simulink model "L400_airframe"  (R2024b)
settings: Solver=FixedStepAuto  StartTime=0  StopTime=10  FixedStep=5/1000  RelTol=1e-3
values from neighbouring files (symbols this model uses):
  db =     [L400_airframe_data.mat]
undefined symbols (not defined in the file or in its folder): lambda
libraries: aerolibconvert2 x16, simulink x6, matrix_library x4, aerolibactuator x2, shared6dof x1, aerolibtransform2 x1
(part 1 of 4)
settings Model: DataDictionary=nextpilot_datadict.sldd  PauseTimes=10  Creator=zhanfuyu  LastModifiedBy=CETCA
settings OptimizationCC: BlockReduction=off  OptimizeBlockIOStorage=off  BufferReuse=off  ReuseModelBlockBuffer=off
settings DebuggingCC: AlgebraicLoopMsg=none
settings RTWCC: GPUComputeCapability=3.5

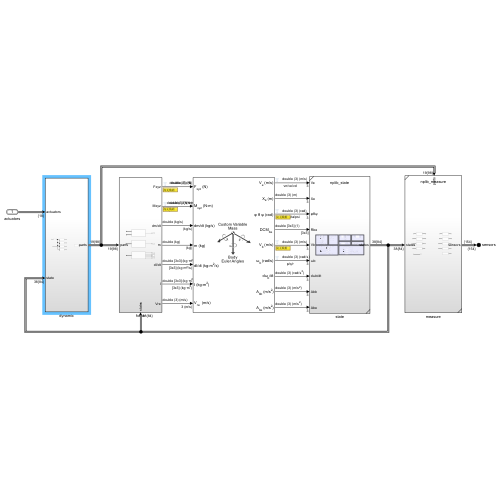
[thumbnail: Simulink's stored preview of the top-level diagram]
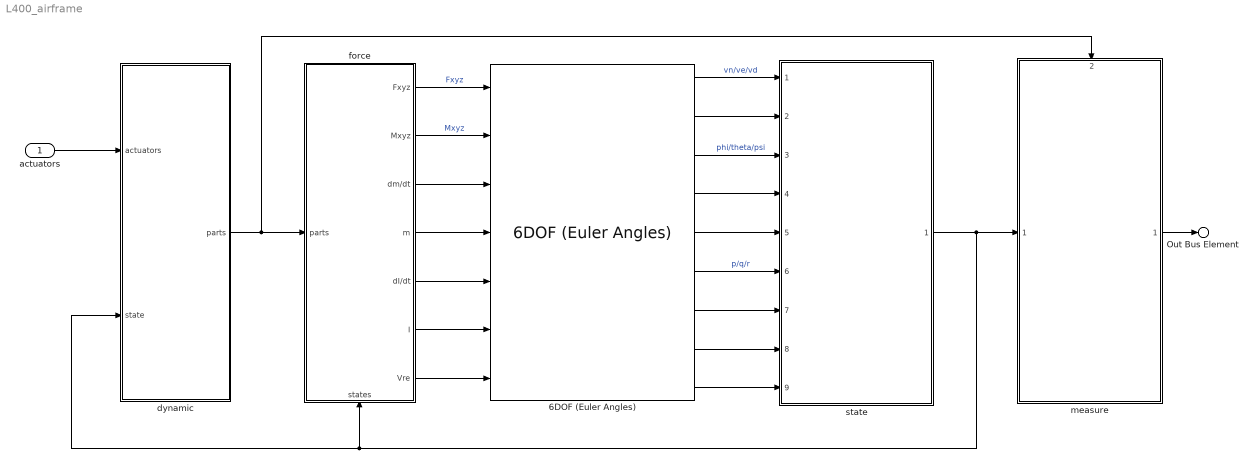
== system L400_airframe ==
  actuators : Inport  OutDataTypeStr=Bus: actuator_outputs_s
  6DOF (Euler Angles) : shared6dof/6DOF (Euler Angles)  units=Metric (MKS)  mtype=Custom Variable  rep=Euler Angles  xme_0=[0 0 0]  Vm_0=INIT_U_V_W  eul_0=INIT_PHI_THETA_PSI  pm_0=INIT_P_Q_R  mass_0=db.mass.empty_weight  mass_e=0.5  mass_f=2.0  inertia=db.mass.empty_inertia  inertia_e=eye(3)  inertia_f=2*eye(3)  k_quat=1.0  vre_flag=on  abi_flag=on  aMode=0  xme_statename=''  Vm_statename=''  eul_statename=''  quat_statename=''  pm_statename=''  mass_statename=''
  dynamic : Subsystem
  force : Subsystem
      settings: PortSchema="{\"entries\":[{\"content\":{\"sides\":[{\"content\":{\"connectorIds\":[\"In1\"]},\"type\":\"ConnectorPlacement.EquallySpacedRectSide\",\"uuid\":\"0db1562e-dce2-4925-bed5-09f9d5b35c44\"},{\"content\":{\"connectorIds\":[\"Out1\",\"Out2\",\"Out3\",\"Out4\",\"Out5\",\"Out6\",\"Out7\"],\"side\":\"RIGHT\"},\"type\":\"ConnectorPlacement.EquallySpacedRectSide\",\"uuid\":\"7a0bc065-1050-4432-a746-8dc7f5e520af\"},{\"content\":{\"side\":\"TOP\"},\"type\":\"ConnectorPlacement.EquallySpacedRectSide\",\"uuid\":\"d0d45c02-cab6-4ab9-ab13-36238f6ff9ea\"},{\"content\":{\"connectorIds\":[\"In2\"],\"side\":\"BOTTOM\"},\"type\":\"ConnectorPlacement.EquallySpacedRectSide\",\"uuid\":\"de54a8ab-f9a4-4296-8b1a-e4e0d752d409\"}]},\"type\":\"ConnectorPlacement.EquallySpacedConnector\",\"uuid\":\"66df0e54-381c-4367-9374-a8940782ebe2\"}],\"packageUris\":[\"http://schema.mathworks.com/mf0/Connector/R2020b\"],\"version\":\"1.0\"}"
  measure : Subsystem  ReferencedSubsystem=nplib_measure
      settings: PortSchema="{\"entries\":[{\"content\":{\"sides\":[{\"content\":{\"connectorIds\":[\"In1\"]},\"type\":\"ConnectorPlacement.EquallySpacedRectSide\",\"uuid\":\"2aab4ced-4e9b-468f-a65b-188f78e0a938\"},{\"content\":{\"connectorIds\":[\"Out1\"],\"side\":\"RIGHT\"},\"type\":\"ConnectorPlacement.EquallySpacedRectSide\",\"uuid\":\"584354fc-f574-4b95-9f8d-a092ecf8eb84\"},{\"content\":{\"connectorIds\":[\"In2\"],\"side\":\"TOP\"},\"type\":\"ConnectorPlacement.EquallySpacedRectSide\",\"uuid\":\"a8f99752-a379-47dc-8675-e6d7e7135bd2\"}]},\"type\":\"ConnectorPlacement.EquallySpacedConnector\",\"uuid\":\"3b032698-2e8e-44bf-976a-546e344c3b42\"}],\"packageUris\":[\"http://schema.mathworks.com/mf0/Connector/R2020b\"],\"version\":\"1.0\"}"
  state : Subsystem  ReferencedSubsystem=nplib_state
  Out Bus Element : Outport  PortName=sensors
  wires:
  state/1 -> dynamic/2(state), force/2(states), measure/1
  measure/1 -> Out Bus Element/1
  actuators/1 -> dynamic/1(actuators)
  6DOF (Euler Angles)/1 -> state/1  "vn/ve/vd"
  6DOF (Euler Angles)/2 -> state/2
  6DOF (Euler Angles)/3 -> state/3  "phi/theta/psi"
  6DOF (Euler Angles)/4 -> state/4
  6DOF (Euler Angles)/5 -> state/5
  6DOF (Euler Angles)/6 -> state/6  "p/q/r"
  6DOF (Euler Angles)/7 -> state/7
  6DOF (Euler Angles)/8 -> state/8
  dynamic/1(parts) -> measure/2, force/1(parts)
  force/4(m) -> 6DOF (Euler Angles)/4
  force/6(I) -> 6DOF (Euler Angles)/6
  force/3(dm/dt) -> 6DOF (Euler Angles)/3
  force/5(dI/dt) -> 6DOF (Euler Angles)/5
  force/7(Vre) -> 6DOF (Euler Angles)/7
  6DOF (Euler Angles)/9 -> state/9
  force/1(Fxyz) -> 6DOF (Euler Angles)/1  "Fxyz"
  force/2(Mxyz) -> 6DOF (Euler Angles)/2  "Mxyz"

== system L400_airframe/dynamic ==
  Bus Element In1 : Inport  PortName=actuators
  Bus Element In : Inport  Port=2  PortName=state
  " propulsion" : Subsystem
  Subsystem : Subsystem
  aerodynamic : Subsystem
  battery : Subsystem
  landgear : Subsystem  Variant=on  VariantControlMode=label  LabelModeActiveChoice=Simple
  payload : Subsystem
  Bus Element Out : Outport  PortName=parts  Element=aerody
  Bus Element Out1 : Outport  PortName=parts  Element=engine
  Bus Element Out2 : Outport  PortName=parts  Element=landgear
  Bus Element Out3 : Outport  PortName=parts  Element=payload
  Bus Element Out4 : Outport  PortName=parts  Element=battery
  wires:
  Bus Element In1/1 -> Subsystem/1(actuators)
  Subsystem/1(command) -> landgear/1(cmd), payload/1(cmd), " propulsion"/1(cmd), aerodynamic/1(cmd)
  aerodynamic/1(aerody) -> Bus Element Out/1
  " propulsion"/1(engine) -> Bus Element Out1/1
  landgear/1(landgear) -> Bus Element Out2/1
  payload/1(payload) -> Bus Element Out3/1
  battery/1(battery) -> Bus Element Out4/1
  Bus Element In/1 -> landgear/2(state), payload/2(state), aerodynamic/2(state), " propulsion"/2(state)

== system L400_airframe/force ==
  BusElementIn : Inport  PortName=parts
  BusElementIn1 : Inport  PortName=parts
  BusElementIn2 : Inport  PortName=parts
  BusElementIn3 : Inport  Port=2  PortName=states
  Force : Subsystem
  Mass : Subsystem
  Moment : Subsystem
  Fxyz : Outport
  Mxyz : Outport  Port=2
  dm/dt : Outport  Port=3
  m : Outport  Port=4
  dI/dt : Outport  Port=5
  I : Outport  Port=6
  Vre : Outport  Port=7
  wires:
  Force/1(Fxyz) -> Fxyz/1
  BusElementIn/1 -> Force/1(parts)
  BusElementIn1/1 -> Moment/1(parts)
  BusElementIn2/1 -> Mass/1(parts)
  Mass/1(dM/dt) -> dm/dt/1
  Mass/2(M) -> m/1
  Mass/3(dI/dt) -> dI/dt/1
  Mass/4(I) -> I/1
  Mass/5(Vre) -> Vre/1
  Moment/1(Mxyz) -> Mxyz/1
  BusElementIn3/1 -> Force/2(state)

== system L400_airframe/dynamic/ propulsion ==
  Bus Element In : Inport  PortName=cmd  Element=DTLO
  Bus Element In2 : Inport  PortName=cmd  Element=DTLI
  Bus Element In3 : Inport  PortName=cmd  Element=DTRI
  Bus Element In4 : Inport  PortName=cmd  Element=DTRO
  BusElementIn : Inport  Port=2  PortName=state  Element=environ.atmosphere.rho
  BusElementIn1 : Inport  Port=2  PortName=state  Element=aircraft.airdata.vax_vay_vaz
  BusElementIn2 : Inport  Port=2  PortName=state  Element=aircraft.airdata.qbar
  Constant1 : Constant  Value=db.motor.setup_position
  Constant2 : Constant  Value=db.motor.setup_angle
  Constant3 : Constant  Value=db.motor.rotation
  Data Type Conversion : DataTypeConversion  SaturateOnIntegerOverflow=off  RndMeth=Floor
  Dot Product : DotProduct  OutDataTypeStr=Inherit: Inherit via internal rule
  For Each Subsystem : Subsystem  TreatAsAtomicUnit=on
  Gain2 : Gain  Gain=db.aerody.Sref
  Linear Second-Order Actuator : aerolibactuator/Linear Second-Order Actuator  Commented=through  wn_fin=1  z_fin=0.3  fin_act_0=0  fin_act_vel=0
  Mux : Mux
  Product : Product  Inputs=*/
  Signal Specification : SignalSpecification  Unit=m
  Sqrt : Sqrt
  Sum3 : Sum  Inputs=1  CollapseMode=Specified dimension  CollapseDim=2
  Transpose3 : Math  Operator=transpose
  Bus Element Out2 : Outport  PortName=engine  Element=state.rpm
  Bus Element Out3 : Outport  PortName=engine  Element=state.power
  Bus Element Out : Outport  PortName=engine  Element=Fxyz
  Bus Element Out1 : Outport  PortName=engine  Element=Mxyz
  Bus Element Out4 : Outport  PortName=engine  Element=Pxyz
  tag scope: TC=global
  wires:
  Bus Element In3/1 -> Mux/3
  Bus Element In2/1 -> Mux/2
  Bus Element In4/1 -> Mux/4
  Bus Element In/1 -> Mux/1
  Mux/1 -> Data Type Conversion/1
  Constant3/1 -> For Each Subsystem/3(rotation)
  For Each Subsystem/1(thrust) -> Sum3/1, Bus Element Out/1
  For Each Subsystem/2(moment) -> Bus Element Out1/1
  For Each Subsystem/3(power) -> Bus Element Out3/1
  Linear Second-Order Actuator/1 -> For Each Subsystem/1(rpm), Bus Element Out2/1  "rpm"
  Constant1/1 -> Transpose3/1
  BusElementIn/1 -> For Each Subsystem/5(rho)
  BusElementIn1/1 -> For Each Subsystem/4(Va)
  Transpose3/1 -> Signal Specification/1
  Constant2/1 -> For Each Subsystem/2(angle)
  Sum3/1 -> Dot Product/2, Dot Product/1
  Dot Product/1 -> Sqrt/1
  Sqrt/1 -> Product/1
  Product/1 -> [TC]
  BusElementIn2/1 -> Gain2/1
  Gain2/1 -> Product/2
  Data Type Conversion/1 -> Linear Second-Order Actuator/1
  Signal Specification/1 -> Bus Element Out4/1

== system L400_airframe/dynamic/Subsystem ==
  Bus Element In1 : Inport  PortName=actuators  Element=output
  Constant : Constant  Value=false
  Data Type Conversion : DataTypeConversion  SaturateOnIntegerOverflow=off  RndMeth=Floor
  Data Type Conversion1 : DataTypeConversion  SaturateOnIntegerOverflow=off  RndMeth=Floor
  Demux : Demux  Outputs=16
  Bus Element Out1 : Outport  PortName=command  Element=DTLO
  Bus Element Out2 : Outport  PortName=command  Element=DTLI
  Bus Element Out3 : Outport  PortName=command  Element=DTRI
  Bus Element Out4 : Outport  PortName=command  Element=DTRO
  Bus Element Out5 : Outport  PortName=command  Element=DFLO
  Bus Element Out6 : Outport  PortName=command  Element=DFLI
  Bus Element Out7 : Outport  PortName=command  Element=DFRI
  Bus Element Out8 : Outport  PortName=command  Element=DFRO
  Bus Element Out9 : Outport  PortName=command  Element=DAL
  Bus Element Out10 : Outport  PortName=command  Element=DAR
  Bus Element Out11 : Outport  PortName=command  Element=DEL
  Bus Element Out12 : Outport  PortName=command  Element=DEM
  Bus Element Out13 : Outport  PortName=command  Element=DER
  Bus Element Out14 : Outport  PortName=command  Element=DRuder
  Bus Element Out15 : Outport  PortName=command  Element=DBrake
  Bus Element Out16 : Outport  PortName=command  Element=DWheel
  Bus Element Out17 : Outport  PortName=command  Element=Dpayload
  wires:
  Bus Element In1/1 -> Demux/1
  Demux/1 -> Bus Element Out1/1
  Demux/2 -> Bus Element Out2/1
  Demux/3 -> Bus Element Out3/1
  Demux/4 -> Bus Element Out4/1
  Demux/5 -> Bus Element Out5/1
  Demux/6 -> Bus Element Out6/1
  Demux/7 -> Bus Element Out7/1
  Demux/8 -> Bus Element Out8/1
  Demux/9 -> Bus Element Out9/1
  Demux/10 -> Bus Element Out10/1
  Demux/11 -> Bus Element Out11/1
  Demux/12 -> Bus Element Out12/1
  Demux/13 -> Bus Element Out13/1
  Demux/14 -> Bus Element Out14/1
  Demux/15 -> Data Type Conversion1/1
  Demux/16 -> Data Type Conversion/1
  Constant/1 -> Bus Element Out17/1
  Data Type Conversion/1 -> Bus Element Out16/1
  Data Type Conversion1/1 -> Bus Element Out15/1

== system L400_airframe/dynamic/aerodynamic ==
  BusElementIn4 : Inport  PortName=cmd
  Bus Element In1 : Inport  Port=2  PortName=state
  actuator : Subsystem
  aerodynamics : Subsystem
  Bus Element Out1 : Outport  PortName=aerody
  wires:
  BusElementIn4/1 -> actuator/1(command)
  Bus Element In1/1 -> aerodynamics/2(state)
  actuator/1(surface) -> aerodynamics/1(surface)
  aerodynamics/1(aerody) -> Bus Element Out1/1

== system L400_airframe/dynamic/battery ==
  note: 50A放电曲线
  note: 电机的功耗
  Constant : Constant  Value=db.battery.capacity
  Constant1 : Constant  Value=db.battery.other_power
  Constant2 : Constant  Value=0
  Gain : Gain  Gain=1/3600/1000
  Integrator : Integrator
  Polynomial : Polyval  Coefs=db.battery.discharge_curve
  Product : Product  Inputs=/*
  Saturation : Saturate  UpperLimit=db.battery.max_discharge  LowerLimit=0
  Sum : Sum  Inputs=|+-
  Sum1 : Sum  Inputs=|++
  Bus Element Out : Outport  PortName=battery  Element=voltage
  Bus Element Out1 : Outport  PortName=battery  Element=soc
  wires:
  Constant/1 -> Product/1, Sum/1
  Integrator/1 -> Gain/1
  Sum/1 -> Polynomial/1, Product/2
  Product/1 -> Bus Element Out1/1
  Polynomial/1 -> Bus Element Out/1
  Gain/1 -> Saturation/1
  Saturation/1 -> Sum/2
  Constant1/1 -> Sum1/1
  Constant2/1 -> Sum1/2
  Sum1/1 -> Integrator/1

== system L400_airframe/dynamic/landgear ==
  note: 1) Add Subsystem or Model blocks as valid variant choices.
      | 2) You cannot connect blocks at this level. At simulation, connectivity is automatically
      | determined, based on the active variant and port name matching.
  cmd : Inport
  state : Inport  Port=2
  Complete : Subsystem  VariantControl=Complete
  Hold : Subsystem  VariantControl=Hold
  Simple : Subsystem  VariantControl=Simple
  landgear : Outport

== system L400_airframe/dynamic/payload ==
  BusElementIn2 : Inport  PortName=cmd  Element=Dpayload
  BusElementIn : Inport  Port=2  PortName=state  Element=aircraft.attitude.phi_theta_psi
  Angle Conversion : aerolibconvert2/Angle Conversion  IU=rad  OU=deg
  Constant : Constant  Value=db.payload.init_mass
  Constant2 : Constant  Commented=on  Value=db.mass.ref_cog
  Constant3 : Constant  Commented=on  Value=[0 0 0]
  Constant4 : Constant  Value=db.payload.spray_speed
  Constant7 : Constant  Value=0
  Integrator : Integrator  LimitOutput=on  UpperSaturationLimit=db.payload.init_mass  LowerSaturationLimit=0
  Selector : Selector  InputPortWidth=3  IndexOptions=Index vector (dialog)  Indices=2  OutputSizes=1
  Subsystem : Subsystem
  Sum : Sum  Inputs=|+-
  Switch : Switch  Criteria=u2 > Threshold  SaturateOnIntegerOverflow=off  InputSameDT=off
  Bus Element Out : Outport  PortName=payload  Element=Fxyz
  Bus Element Out1 : Outport  PortName=payload  Element=Mxyz
  Bus Element Out2 : Outport  PortName=payload  Element=mass
  Bus Element Out3 : Outport  PortName=payload  Element=inertia
  Bus Element Out4 : Outport  PortName=payload  Element=cog
  Bus Element Out5 : Outport  PortName=payload  Element=Pxyz
  wires:
  Constant2/1 -> Bus Element Out5/1
  Constant3/1 -> Bus Element Out/1, Bus Element Out1/1
  Constant/1 -> Sum/1
  Sum/1 -> Bus Element Out2/1, Subsystem/1(mass)
  BusElementIn/1 -> Selector/1
  Selector/1 -> Angle Conversion/1
  BusElementIn2/1 -> Switch/2
  Constant4/1 -> Switch/1
  Switch/1 -> Integrator/1
  Constant7/1 -> Switch/3
  Integrator/1 -> Sum/2
  Subsystem/2(inertia) -> Bus Element Out3/1
  Angle Conversion/1 -> Subsystem/2(theta)
  Subsystem/1(cog) -> Bus Element Out4/1

== system L400_airframe/force/Force ==
  BusElementIn1 : Inport  PortName=parts  Element=aerody.Fxyz
  BusElementIn2 : Inport  PortName=parts  Element=engine.Fxyz
  BusElementIn3 : Inport  PortName=parts  Element=landgear.Fxyz
  BusElementIn4 : Inport  Port=2  PortName=state  Element=environ.gravity.gx_gy_gz
  Product : Product
  Reshape : Reshape
  Reshape1 : Reshape
  Sum : Sum  Inputs=4
  Sum1 : Sum  Inputs=1  CollapseMode=Specified dimension  CollapseDim=2
  Sum2 : Sum  Inputs=+-|
  Sum3 : Sum  Inputs=1  CollapseMode=Specified dimension  CollapseDim=2
  Fxyz : Outport
  tag scope: Fxyz_no_ground=global
  wires:
  BusElementIn2/1 -> Sum3/1
  BusElementIn1/1 -> Sum/2
  Sum/1 -> Sum2/1, Fxyz/1
  [mass] -> Product/1
  Sum3/1 -> Reshape/1
  Reshape/1 -> Sum/3
  BusElementIn3/1 -> Sum1/1
  BusElementIn4/1 -> Product/2
  Sum1/1 -> Reshape1/1
  Reshape1/1 -> Sum/4, Sum2/2
  Product/1 -> Sum/1
  Sum2/1 -> [Fxyz_no_ground]

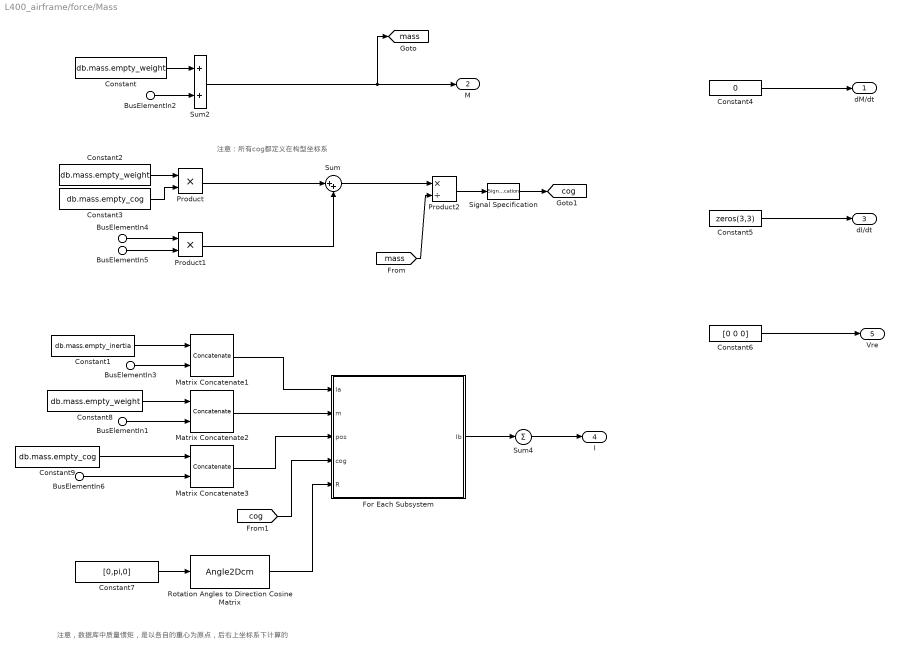
== system L400_airframe/force/Mass ==
  note: 注意，数据库中质量惯矩，是以各自的重心为原点，后右上坐标系下计算的
  note: 注意：所有cog都定义在构型坐标系
  BusElementIn3 : Inport  PortName=parts  Element=payload.inertia
  BusElementIn5 : Inport  PortName=parts  Element=payload.cog
  BusElementIn6 : Inport  PortName=parts  Element=payload.cog
  BusElementIn2 : Inport  PortName=parts  Element=payload.mass
  BusElementIn4 : Inport  PortName=parts  Element=payload.mass
  BusElementIn1 : Inport  PortName=parts  Element=payload.mass
  Constant : Constant  Value=db.mass.empty_weight
  Constant1 : Constant  Value=db.mass.empty_inertia
  Constant2 : Constant  Value=db.mass.empty_weight
  Constant3 : Constant  Value=db.mass.empty_cog
  Constant4 : Constant  Value=0
  Constant5 : Constant  Value=zeros(3,3)
  Constant6 : Constant  Value=[0 0 0]
  Constant7 : Constant  Value=[0,pi,0]
  Constant8 : Constant  Value=db.mass.empty_weight
  Constant9 : Constant  Value=db.mass.empty_cog
  For Each Subsystem : Subsystem  TreatAsAtomicUnit=on
  Matrix Concatenate1 : Concatenate  Mode=Multidimensional array  ConcatenateDimension=3
  Matrix Concatenate2 : Concatenate  Mode=Multidimensional array  ConcatenateDimension=3
  Matrix Concatenate3 : Concatenate  Mode=Multidimensional array  ConcatenateDimension=3
  Product : Product
  Product1 : Product
  Product2 : Product  Inputs=*/
  Rotation Angles to Direction Cosine Matrix : Angle2Dcm
      settings: AttributesFormatString=Rotation Order: %<rotationOrder>
  Signal Specification : SignalSpecification  Unit=m
  Sum : Sum  Inputs=|++
  Sum2 : Sum  Inputs=2
  Sum4 : Sum  Inputs=1  CollapseMode=Specified dimension  CollapseDim=3
  dM/dt : Outport
  M : Outport  Port=2
  dI/dt : Outport  Port=3
  I : Outport  Port=4
  Vre : Outport  Port=5
  tag scope: cog=global, mass=global
  wires:
  Product1/1 -> Sum/2
  Constant3/1 -> Product/2
  BusElementIn5/1 -> Product1/2
  Product/1 -> Sum/1
  [mass] -> Product2/2
  BusElementIn4/1 -> Product1/1
  Sum/1 -> Product2/1
  Constant2/1 -> Product/1
  Product2/1 -> Signal Specification/1
  BusElementIn2/1 -> Sum2/2
  Constant/1 -> Sum2/1
  Constant4/1 -> dM/dt/1
  Constant5/1 -> dI/dt/1
  Constant6/1 -> Vre/1
  Constant7/1 -> Rotation Angles to Direction Cosine Matrix/1
  [cog] -> For Each Subsystem/4(cog)
  Constant1/1 -> Matrix Concatenate1/1
  BusElementIn3/1 -> Matrix Concatenate1/2
  Matrix Concatenate1/1 -> For Each Subsystem/1(Ia)
  Matrix Concatenate2/1 -> For Each Subsystem/2(m)
  BusElementIn1/1 -> Matrix Concatenate2/2
  Constant8/1 -> Matrix Concatenate2/1
  Matrix Concatenate3/1 -> For Each Subsystem/3(pos)
  Rotation Angles to Direction Cosine Matrix/1 -> For Each Subsystem/5(R)
  BusElementIn6/1 -> Matrix Concatenate3/2
  Sum4/1 -> I/1
  Constant9/1 -> Matrix Concatenate3/1
  For Each Subsystem/1(Ib) -> Sum4/1
  Sum2/1 -> M/1, [mass]
  Signal Specification/1 -> [cog]

== system L400_airframe/force/Moment ==
  BusElementIn : Inport  PortName=parts  Element=aerody.Mxyz
  BusElementIn3 : Inport  PortName=parts  Element=aerody.Fxyz
  BusElementIn8 : Inport  PortName=parts  Element=aerody.Pxyz
  BusElementIn2 : Inport  PortName=parts  Element=engine.Mxyz
  BusElementIn5 : Inport  PortName=parts  Element=engine.Fxyz
  BusElementIn7 : Inport  PortName=parts  Element=engine.Pxyz
  BusElementIn1 : Inport  PortName=parts  Element=landgear.Mxyz
  BusElementIn4 : Inport  PortName=parts  Element=landgear.Fxyz
  BusElementIn6 : Inport  PortName=parts  Element=landgear.Pxyz
  For Each Subsystem : Subsystem  TreatAsAtomicUnit=on
  Matrix Concatenate : Concatenate  NumInputs=3  Mode=Multidimensional array  ConcatenateDimension=2
  Matrix Concatenate1 : Concatenate  NumInputs=3  Mode=Multidimensional array  ConcatenateDimension=2
  Matrix Concatenate2 : Concatenate  NumInputs=3  Mode=Multidimensional array  ConcatenateDimension=2
  Reshape : Reshape
  Reshape1 : Reshape
  Selector : Selector  NumberOfDimensions=2  InputPortWidth=3  IndexOptions=Select all,Index vector (dialog)  Indices=[1 3],1:5  OutputSizes=1,1
  Signal Specification : SignalSpecification  Dimensions=3
  Signal Specification1 : SignalSpecification  Dimensions=3
  Sum : Sum  Inputs=1  CollapseMode=Specified dimension  CollapseDim=2
  Sum1 : Sum  Inputs=1  CollapseMode=Specified dimension  CollapseDim=2
  Mxyz : Outport
  tag scope: Mxyz_no_ground=global
  wires:
  BusElementIn3/1 -> Signal Specification/1
  Signal Specification/1 -> Matrix Concatenate/1
  BusElementIn5/1 -> Matrix Concatenate/2
  BusElementIn4/1 -> Matrix Concatenate/3
  Matrix Concatenate/1 -> For Each Subsystem/1(Fxyz)
  BusElementIn2/1 -> Matrix Concatenate1/2
  BusElementIn1/1 -> Matrix Concatenate1/3
  BusElementIn/1 -> Signal Specification1/1
  Matrix Concatenate1/1 -> For Each Subsystem/2(Mxyz)
  Matrix Concatenate2/1 -> For Each Subsystem/3(Pxyz)
  BusElementIn7/1 -> Matrix Concatenate2/2
  BusElementIn6/1 -> Matrix Concatenate2/3
  BusElementIn8/1 -> Matrix Concatenate2/1
  [cog] -> For Each Subsystem/4(COG)
  Sum/1 -> Reshape/1
  Reshape/1 -> Mxyz/1
  Signal Specification1/1 -> Matrix Concatenate1/1
  For Each Subsystem/1(M) -> Selector/1, Sum/1
  Sum1/1 -> Reshape1/1
  Reshape1/1 -> [Mxyz_no_ground]
  Selector/1 -> Sum1/1

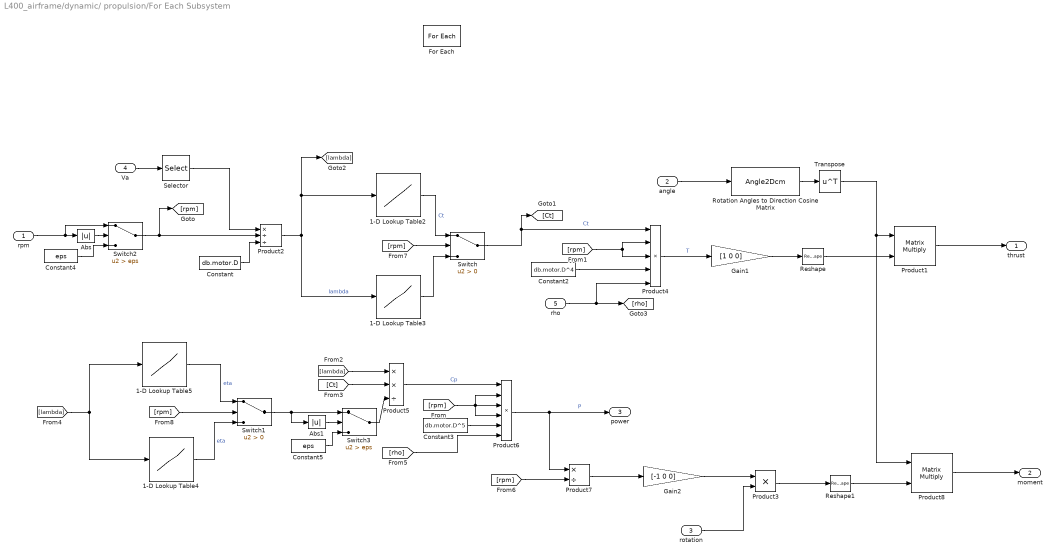
== system L400_airframe/dynamic/ propulsion/For Each Subsystem ==
  rpm : Inport  Unit=rad/s  Partition=on  PartitionDimension=1  PartitionWidth=1  PartitionOffset=0
  angle : Inport  Port=2  Unit=rad  Partition=on  PartitionDimension=1  PartitionWidth=1  PartitionOffset=0
  rotation : Inport  Port=3  Partition=on  PartitionDimension=1  PartitionWidth=1  PartitionOffset=0
  Va : Inport  Port=4  Unit=m/s
  rho : Inport  Port=5
  1-D Lookup Table2 : Lookup_n-D  NumberOfTableDimensions=1  BreakpointsForDimension1=db.motor.lambda  IndexSearchMethod=Linear search  BeginIndexSearchUsingPreviousIndexResult=on  Table=db.motor.Ct  ExtrapMethod=Clip  InternalRulePriority=Speed  RndMeth=Simplest
  1-D Lookup Table3 : Lookup_n-D  NumberOfTableDimensions=1  BreakpointsForDimension1=db.motor.lambda_rev  IndexSearchMethod=Linear search  BeginIndexSearchUsingPreviousIndexResult=on  Table=db.motor.Ct_rev  ExtrapMethod=Clip  InternalRulePriority=Speed  RndMeth=Simplest
  1-D Lookup Table4 : Lookup_n-D  NumberOfTableDimensions=1  BreakpointsForDimension1=db.motor.lambda_rev  IndexSearchMethod=Linear search  BeginIndexSearchUsingPreviousIndexResult=on  Table=db.motor.eta_rev  ExtrapMethod=Clip  InternalRulePriority=Speed  RndMeth=Simplest
  1-D Lookup Table5 : Lookup_n-D  NumberOfTableDimensions=1  BreakpointsForDimension1=db.motor.lambda  IndexSearchMethod=Linear search  BeginIndexSearchUsingPreviousIndexResult=on  Table=db.motor.eta  ExtrapMethod=Clip  InternalRulePriority=Speed  RndMeth=Simplest
  Abs : Abs  SaturateOnIntegerOverflow=off
  Abs1 : Abs  SaturateOnIntegerOverflow=off
  Constant : Constant  Value=db.motor.D
  Constant2 : Constant  Value=db.motor.D^4
  Constant3 : Constant  Value=db.motor.D^5
  Constant4 : Constant  Value=eps
  Constant5 : Constant  Value=eps
  For Each : ForEach  DisableCoverage=on
  Gain1 : Gain  Gain=[1 0 0]
  Gain2 : Gain  Gain=[-1 0 0]
  Product1 : Product  Multiplication=Matrix(*)
  Product2 : Product  Inputs=*//
  Product3 : Product
  Product4 : Product  Inputs=5
  Product5 : Product  Inputs=**/
  Product6 : Product  Inputs=6
  Product7 : Product  Inputs=*/
  Product8 : Product  Multiplication=Matrix(*)
  Reshape : Reshape  OutputDimensionality=Column vector (2-D)
  Reshape1 : Reshape  OutputDimensionality=Column vector (2-D)
  Rotation Angles to Direction Cosine Matrix : Angle2Dcm
      settings: AttributesFormatString=Rotation Order: %<rotationOrder>
  Selector : Selector  InputPortWidth=3  IndexOptions=Index vector (dialog)  Indices=1  OutputSizes=1
  Switch : Switch  Criteria=u2 > Threshold  SaturateOnIntegerOverflow=off  InputSameDT=off
  Switch1 : Switch  Criteria=u2 > Threshold  SaturateOnIntegerOverflow=off  InputSameDT=off
  Switch2 : Switch  Criteria=u2 > Threshold  Threshold=eps  SaturateOnIntegerOverflow=off  InputSameDT=off
  Switch3 : Switch  Criteria=u2 > Threshold  Threshold=eps  SaturateOnIntegerOverflow=off  InputSameDT=off
  Transpose : Math  Operator=transpose
  thrust : Outport  Unit=N  ConcatenationDimension=2
  moment : Outport  Port=2  Unit=N*m  ConcatenationDimension=2
  power : Outport  Port=3  Unit=W  ConcatenationDimension=1
  wires:
  angle/1 -> Rotation Angles to Direction Cosine Matrix/1
  Rotation Angles to Direction Cosine Matrix/1 -> Transpose/1
  Transpose/1 -> Product8/1, Product1/1
  Product1/1 -> thrust/1
  Product3/1 -> Reshape1/1
  Switch/1 -> [Ct], Product4/1  "Ct"
  Va/1 -> Selector/1
  rpm/1 -> Abs/1, Switch2/1
  Product2/1 -> 1-D Lookup Table2/1, [lambda], 1-D Lookup Table3/1  "lambda"
  Constant/1 -> Product2/3
  rho/1 -> [rho], Product4/5
  Product4/1 -> Gain1/1  "T"
  1-D Lookup Table5/1 -> Switch1/1  "eta"
  Product5/1 -> Product6/1  "Cp"
  [rpm] -> Product4/3, Product4/2
  Constant2/1 -> Product4/4
  [lambda] -> Product5/1
  [Ct] -> Product5/2
  [lambda] -> 1-D Lookup Table5/1, 1-D Lookup Table4/1
  [rpm] -> Product6/2, Product6/4, Product6/3
  Constant3/1 -> Product6/5
  [rho] -> Product6/6
  Product6/1 -> Product7/1, power/1  "P"
  [rpm] -> Product7/2
  Product7/1 -> Gain2/1
  Selector/1 -> Product2/1
  1-D Lookup Table2/1 -> Switch/1  "Ct"
  [rpm] -> Switch/2
  1-D Lookup Table3/1 -> Switch/3
  [rpm] -> Switch1/2
  1-D Lookup Table4/1 -> Switch1/3  "eta"
  Gain1/1 -> Reshape/1
  Switch2/1 -> [rpm], Product2/2
  Constant4/1 -> Switch2/3
  Constant5/1 -> Switch3/3
  Switch1/1 -> Abs1/1, Switch3/1
  Switch3/1 -> Product5/3
  Abs/1 -> Switch2/2
  Abs1/1 -> Switch3/2
  Reshape/1 -> Product1/2
  Gain2/1 -> Product3/1
  rotation/1 -> Product3/2
  Reshape1/1 -> Product8/2
  Product8/1 -> moment/1

== system L400_airframe/dynamic/aerodynamic/actuator ==
  BusElementIn1 : Inport  PortName=command  Element=DAL
  BusElementIn2 : Inport  PortName=command  Element=DER
  BusElementIn3 : Inport  PortName=command  Element=DRuder
  BusElementIn4 : Inport  PortName=command  Element=DEM
  BusElementIn5 : Inport  PortName=command  Element=DEL
  BusElementIn6 : Inport  PortName=command  Element=DFLO
  BusElementIn7 : Inport  PortName=command  Element=DFLI
  BusElementIn8 : Inport  PortName=command  Element=DFRI
  BusElementIn9 : Inport  PortName=command  Element=DFRO
  BusElementIn : Inport  PortName=command  Element=DAR
  Data Type Conversion : DataTypeConversion  SaturateOnIntegerOverflow=off  RndMeth=Floor
  Demux : Demux  Outputs=10
  Mux : Mux  Inputs=10
  Saturation : Saturate  UpperLimit=[30,30,30,30,15,15,17,17,17,23]  LowerLimit=[0,0,0,0,-23,-23,-23,-23,-23,-23]
  Signal Specification4 : SignalSpecification  Unit=deg
  Variant Subsystem : Subsystem  Variant=on
  Bus Element Out : Outport  PortName=surface  Element=DFLO
  Bus Element Out1 : Outport  PortName=surface  Element=DFLI
  Bus Element Out2 : Outport  PortName=surface  Element=DFRI
  Bus Element Out3 : Outport  PortName=surface  Element=DFRO
  Bus Element Out4 : Outport  PortName=surface  Element=DAL
  Bus Element Out5 : Outport  PortName=surface  Element=DAR
  Bus Element Out6 : Outport  PortName=surface  Element=DEL
  Bus Element Out7 : Outport  PortName=surface  Element=DEM
  Bus Element Out8 : Outport  PortName=surface  Element=DER
  Bus Element Out9 : Outport  PortName=surface  Element=DR
  wires:
  Mux/1 -> Data Type Conversion/1
  Saturation/1 -> Signal Specification4/1
  Variant Subsystem/1(Out1) -> Demux/1
  Demux/1 -> Bus Element Out/1
  Demux/2 -> Bus Element Out1/1
  Demux/4 -> Bus Element Out3/1
  Demux/3 -> Bus Element Out2/1
  Signal Specification4/1 -> Variant Subsystem/1(In1)
  BusElementIn6/1 -> Mux/1
  BusElementIn7/1 -> Mux/2
  BusElementIn8/1 -> Mux/3
  BusElementIn9/1 -> Mux/4
  BusElementIn3/1 -> Mux/10
  BusElementIn2/1 -> Mux/9
  BusElementIn5/1 -> Mux/7
  BusElementIn4/1 -> Mux/8
  BusElementIn/1 -> Mux/6
  BusElementIn1/1 -> Mux/5
  Demux/5 -> Bus Element Out4/1
  Demux/6 -> Bus Element Out5/1
  Demux/7 -> Bus Element Out6/1
  Demux/8 -> Bus Element Out7/1
  Demux/9 -> Bus Element Out8/1
  Demux/10 -> Bus Element Out9/1
  Data Type Conversion/1 -> Saturation/1

== system L400_airframe/dynamic/aerodynamic/aerodynamics ==
  note: 当前向空速小于3m/s的时候，此时迎角侧滑角都不准却，因此禁用空气动力
  BusElementIn7 : Inport  PortName=surface
  BusElementIn9 : Inport  Port=2  PortName=state
  BusElementIn : Inport  Port=2  PortName=state  Element=aircraft.airdata.vax_vay_vaz
  Abs : Abs  SaturateOnIntegerOverflow=off
  If : If  IfExpression=u1 > 3
  If Action Subsystem : Subsystem  TreatAsAtomicUnit=on
  If Action Subsystem1 : Subsystem  TreatAsAtomicUnit=on
  Merge : Merge
  Selector : Selector  InputPortWidth=3  IndexOptions=Index vector (dialog)  Indices=1  OutputSizes=1
  Bus Element Out : Outport  PortName=aerody
  wires:
  BusElementIn/1 -> Selector/1
  Abs/1 -> If/1
  If/1 -> If Action Subsystem/Action
  If/2 -> If Action Subsystem1/Action
  BusElementIn7/1 -> If Action Subsystem/1(surface)
  BusElementIn9/1 -> If Action Subsystem/2(state)
  If Action Subsystem/1(aerody) -> Merge/1
  If Action Subsystem1/1(aerody) -> Merge/2
  Merge/1 -> Bus Element Out/1
  [TC] -> If Action Subsystem/3(TC)

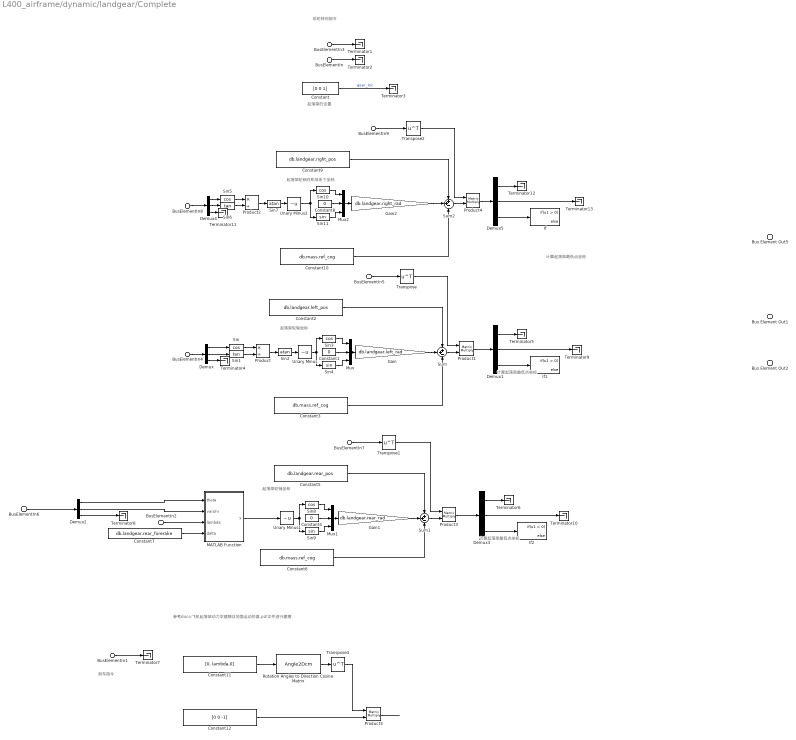
== system L400_airframe/dynamic/landgear/Complete ==
  note: 起落架轮轴坐标
  note: 计算起落架最低点坐标
  note: 刹车指令
  note: 起落架的位置
  note: 后轮转向指令
  note: 起落架轮轴坐标
  note: 计算起落架最低点坐标
  note: 起落架轮轴在机体系下坐标
  note: 计算起落架最低点坐标
  note: 参考docs/飞机起落架动力学建模及地面运动仿真.pdf文件进行建模
  BusElementIn1 : Inport  PortName=cmd  Element=DBrake
  BusElementIn2 : Inport  PortName=cmd  Element=DWheel
  BusElementIn : Inport  Port=2  PortName=state  Element=aircraft.position.agl
  BusElementIn3 : Inport  Port=2  PortName=state  Element=aircraft.position.alt
  BusElementIn4 : Inport  Port=2  PortName=state  Element=aircraft.attitude.phi_theta_psi
  BusElementIn6 : Inport  Port=2  PortName=state  Element=aircraft.attitude.phi_theta_psi
  BusElementIn8 : Inport  Port=2  PortName=state  Element=aircraft.attitude.phi_theta_psi
  BusElementIn5 : Inport  Port=2  PortName=state  Element=aircraft.attitude.Rbe
  BusElementIn7 : Inport  Port=2  PortName=state  Element=aircraft.attitude.Rbe
  BusElementIn9 : Inport  Port=2  PortName=state  Element=aircraft.attitude.Rbe
  Constant : Constant  Value=[0 0 1]
  Constant1 : Constant  Value=0
  Constant10 : Constant  Value=db.mass.ref_cog
  Constant11 : Constant  Value=[0, lambda,0]
  Constant12 : Constant  Value=[0 0 -1]
  Constant2 : Constant  Value=db.landgear.left_pos
  Constant3 : Constant  Value=db.mass.ref_cog
  Constant4 : Constant  Value=0
  Constant5 : Constant  Value=db.landgear.rear_pos
  Constant6 : Constant  Value=db.mass.ref_cog
  Constant7 : Constant  Value=db.landgear.rear_forerake
  Constant8 : Constant  Value=0
  Constant9 : Constant  Value=db.landgear.right_pos
  Demux : Demux  Outputs=3
  Demux1 : Demux  Outputs=[1,2,3]
  Demux2 : Demux  Outputs=3
  Demux3 : Demux  Outputs=[1,2,3]
  Demux4 : Demux  Outputs=3
  Demux5 : Demux  Outputs=[1,2,3]
  Gain : Gain  Gain=db.landgear.left_rad
  Gain1 : Gain  Gain=db.landgear.rear_rad
  Gain2 : Gain  Gain=db.landgear.right_rad
  If : If
  If1 : If
  If2 : If
  MATLAB Function : MATLAB Function  TreatAsAtomicUnit=on
  Mux : Mux  Inputs=3
  Mux1 : Mux  Inputs=3
  Mux2 : Mux  Inputs=3
  Product : Product  Inputs=*/
  Product{1,3..5} (4 alike) : Product  Multiplication=Matrix(*)
  Product2 : Product  Inputs=*/
  Rotation Angles to Direction Cosine Matrix : Angle2Dcm
      settings: AttributesFormatString=Rotation Order: %<rotationOrder>
  Sin{,3,5,8,10} (5 alike) : Trigonometry  Operator=cos
  Sin1 : Trigonometry  Operator=tan
  Sin11 : Trigonometry
  Sin2 : Trigonometry  Operator=atan
  Sin4 : Trigonometry
  Sin6 : Trigonometry  Operator=tan
  Sin7 : Trigonometry  Operator=atan
  Sin9 : Trigonometry
  Sum : Sum  Inputs=++-
  Sum1 : Sum  Inputs=++-
  Sum2 : Sum  Inputs=++-
  Terminator{1..13} (13 alike) : Terminator
  Transpose{,1..3} (4 alike) : Math  Operator=transpose
  Unary Minus : UnaryMinus
  Unary Minus1 : UnaryMinus
  Unary Minus2 : UnaryMinus
  Bus Element Out5 : Outport  PortName=landgear  Element=Fxyz
  Bus Element Out1 : Outport  PortName=landgear  Element=Mxyz
  Bus Element Out2 : Outport  PortName=landgear  Element=Pxyz
  wires:
  Constant/1 -> Terminator3/1  "gear_loc"
  BusElementIn1/1 -> Terminator7/1
  BusElementIn3/1 -> Terminator1/1
  BusElementIn/1 -> Terminator2/1
  BusElementIn4/1 -> Demux/1
  Demux/2 -> Sin1/1
  Demux/1 -> Sin/1
  Sin/1 -> Product/1
  Sin1/1 -> Product/2
  Product/1 -> Sin2/1
  Demux/3 -> Terminator4/1
  Sin2/1 -> Unary Minus/1
  Constant1/1 -> Mux/2
  Sin3/1 -> Mux/1
  Sin4/1 -> Mux/3
  Mux/1 -> Gain/1
  BusElementIn5/1 -> Transpose/1
  Transpose/1 -> Product1/1
  Sum/1 -> Product1/2
  Unary Minus/1 -> Sin4/1, Sin3/1
  Constant2/1 -> Sum/1
  Gain/1 -> Sum/2
  Constant3/1 -> Sum/3
  Constant6/1 -> Sum1/3
  Gain1/1 -> Sum1/2
  Constant5/1 -> Sum1/1
  Unary Minus1/1 -> Sin8/1, Sin9/1
  Sum1/1 -> Product3/2
  Transpose1/1 -> Product3/1
  BusElementIn7/1 -> Transpose1/1
  Mux1/1 -> Gain1/1
  Sin9/1 -> Mux1/3
  Sin8/1 -> Mux1/1
  Constant4/1 -> Mux1/2
  MATLAB Function/1(y) -> Unary Minus1/1
  Demux2/3 -> Terminator8/1
  Demux2/1 -> MATLAB Function/1(theta)
  Demux2/2 -> MATLAB Function/2(varphi)
  BusElementIn6/1 -> Demux2/1
  BusElementIn2/1 -> MATLAB Function/3(lambda)
  Constant7/1 -> MATLAB Function/4(delta)
  Demux5/2 -> Terminator13/1
  Demux5/1 -> Terminator12/1
  Product4/1 -> Demux5/1
  Constant10/1 -> Sum2/3
  Gain2/1 -> Sum2/2
  Constant9/1 -> Sum2/1
  Unary Minus2/1 -> Sin10/1, Sin11/1
  Sum2/1 -> Product4/2
  Transpose2/1 -> Product4/1
  BusElementIn9/1 -> Transpose2/1
  Mux2/1 -> Gain2/1
  Sin11/1 -> Mux2/3
  Sin10/1 -> Mux2/1
  Constant8/1 -> Mux2/2
  Sin7/1 -> Unary Minus2/1
  Demux4/3 -> Terminator11/1
  Product2/1 -> Sin7/1
  Sin6/1 -> Product2/2
  Sin5/1 -> Product2/1
  Demux4/1 -> Sin5/1
  Demux4/2 -> Sin6/1
  BusElementIn8/1 -> Demux4/1
  Demux5/3 -> If/1
  Demux1/3 -> If1/1
  Product1/1 -> Demux1/1
  Demux1/1 -> Terminator5/1
  Demux1/2 -> Terminator9/1
  Demux3/2 -> Terminator10/1
  Demux3/1 -> Terminator6/1
  Demux3/3 -> If2/1
  Product3/1 -> Demux3/1
  Constant11/1 -> Rotation Angles to Direction Cosine Matrix/1
  Rotation Angles to Direction Cosine Matrix/1 -> Transpose3/1
  Constant12/1 -> Product5/2
  Transpose3/1 -> Product5/1
  Product5/1 -> ?
  ? -> Bus Element Out5/1
  ? -> Bus Element Out2/1
  ? -> Bus Element Out1/1

== system L400_airframe/dynamic/landgear/Hold ==
  BusElementIn : Inport  PortName=cmd
  BusElementIn2 : Inport  Port=2  PortName=state  Element=aircraft.position.vn_ve_vd
  BusElementIn3 : Inport  Port=2  PortName=state  Element=aircraft.position.agl
  BusElementIn4 : Inport  Port=2  PortName=state  Element=aircraft.attitude.phi_theta_psi
  BusElementIn5 : Inport  Port=2  PortName=state  Element=aircraft.attitude.p_q_r
  Constant1 : Constant  Value=db.mass.ref_cog
  Constant3 : Constant  Value=[0 0 0]
  Gain : Gain  Gain=1e5
  Gain1 : Gain  Gain=-1e4
  Gain2 : Gain  Gain=[0 0 1]
  Gain3 : Gain  Gain=-5e4
  Gain4 : Gain  Gain=-2e3
  Matrix Concatenate1 : Concatenate  NumInputs=3  Mode=Multidimensional array  ConcatenateDimension=2
  Matrix Concatenate2 : Concatenate  NumInputs=3  Mode=Multidimensional array  ConcatenateDimension=2
  Matrix Concatenate3 : Concatenate  NumInputs=3  Mode=Multidimensional array  ConcatenateDimension=2
  Sum : Sum  Inputs=|++
  Sum1 : Sum  Inputs=|++
  Switch{,1..3} (4 alike) : Switch  Criteria=u2 > Threshold  SaturateOnIntegerOverflow=off  InputSameDT=off
  Terminator : Terminator
  Bus Element Out5 : Outport  PortName=landgear  Element=Fxyz
  Bus Element Out1 : Outport  PortName=landgear  Element=Mxyz
  Bus Element Out2 : Outport  PortName=landgear  Element=Pxyz
  wires:
  BusElementIn3/1 -> Switch/2, Gain2/1, Switch1/2, Switch2/2, Switch3/2
  Gain4/1 -> Sum1/2
  Gain/1 -> Sum/1
  Switch3/1 -> Gain4/1
  Gain2/1 -> Switch/3
  BusElementIn5/1 -> Switch3/3
  BusElementIn2/1 -> Switch1/3
  BusElementIn4/1 -> Switch2/3
  Constant3/1 -> Switch3/1, Switch2/1, Switch1/1, Switch/1
  Switch1/1 -> Gain1/1
  Gain1/1 -> Sum/2
  Switch/1 -> Gain/1
  Gain3/1 -> Sum1/1
  Switch2/1 -> Gain3/1
  BusElementIn/1 -> Terminator/1
  Constant1/1 -> Matrix Concatenate1/2, Matrix Concatenate1/1, Matrix Concatenate1/3
  Matrix Concatenate1/1 -> Bus Element Out2/1
  Sum1/1 -> Matrix Concatenate2/1, Matrix Concatenate2/3, Matrix Concatenate2/2
  Matrix Concatenate2/1 -> Bus Element Out1/1
  Sum/1 -> Matrix Concatenate3/1, Matrix Concatenate3/3, Matrix Concatenate3/2
  Matrix Concatenate3/1 -> Bus Element Out5/1

== system L400_airframe/dynamic/landgear/Simple ==
  cmd : Inport
  state : Inport  Port=2
  Matrix Concatenate : Concatenate  NumInputs=3  Mode=Multidimensional array  ConcatenateDimension=2
  Matrix Concatenate1 : Concatenate  NumInputs=3  Mode=Multidimensional array  ConcatenateDimension=2
  Matrix Concatenate2 : Concatenate  NumInputs=3  Mode=Multidimensional array  ConcatenateDimension=2
  ground static friction : Subsystem
  left : Subsystem
  rear : Subsystem
  right : Subsystem
  Bus Element Out5 : Outport  PortName=landgear  Element=Fxyz
  Bus Element Out1 : Outport  PortName=landgear  Element=Mxyz
  Bus Element Out2 : Outport  PortName=landgear  Element=Pxyz
  wires:
  cmd/1 -> right/1(cmd), left/1(cmd), rear/1(cmd)
  state/1 -> right/2(state), left/2(state), rear/2(state)
  left/1(Fxyz) -> Matrix Concatenate1/2
  rear/1(Fxyz) -> Matrix Concatenate1/1
  right/1(Fxyz) -> Matrix Concatenate1/3
  Matrix Concatenate1/1 -> Bus Element Out5/1
  Matrix Concatenate2/1 -> Bus Element Out1/1
  Matrix Concatenate/1 -> Bus Element Out2/1
  rear/2(Mxyz) -> Matrix Concatenate2/1
  left/2(Mxyz) -> Matrix Concatenate2/2
  right/2(Mxyz) -> Matrix Concatenate2/3
  rear/3(Pxyz) -> Matrix Concatenate/1
  left/3(Pxyz) -> Matrix Concatenate/2
  right/3(Pxyz) -> Matrix Concatenate/3
  ground static friction/1(rear) -> rear/3(param)
  ground static friction/2(left) -> left/3(param)
  ground static friction/3(right) -> right/3(param)
  [cog] -> right/4(cog), left/4(cog), rear/4(cog)

== system L400_airframe/dynamic/payload/Subsystem ==
  note: 注意catia计算的Ixy等已经添加了负号
      | % I = [
      | % Ixx, -Ixy, -Ixz
      | % -Iyx, Iyy, -Iyz
      | % -Izx, -Izy, Izz
      | % ]
  mass : Inport
  theta : Inport  Port=2
  Constant8 : Constant  Value=db.payload.cog
  Constant9 : Constant  Value=db.payload.inertia
  Demux : Demux  Outputs=[3 6]
  Demux1 : Demux  Outputs=6
  For Each Subsystem : Subsystem  TreatAsAtomicUnit=on
  Matrix Concatenate1 : Concatenate  Mode=Multidimensional array  ConcatenateDimension=3
  Mux : Mux  Inputs=9
  Reshape : Reshape  OutputDimensionality=Customize  OutputDimensions=[3 3]
  cog : Outport
  inertia : Outport  Port=2
  wires:
  Matrix Concatenate1/1 -> For Each Subsystem/3(table)
  theta/1 -> For Each Subsystem/2(theta)
  mass/1 -> For Each Subsystem/1(mass)
  Constant9/1 -> Matrix Concatenate1/2
  Constant8/1 -> Matrix Concatenate1/1
  For Each Subsystem/1(interp) -> Demux/1
  Demux/1 -> cog/1
  Demux/2 -> Demux1/1
  Demux1/1 -> Mux/1  "Ixx"
  Demux1/2 -> Mux/5  "Iyy"
  Demux1/3 -> Mux/9  "Izz"
  Demux1/4 -> Mux/4, Mux/2  "Ixy"
  Demux1/5 -> Mux/3, Mux/7  "Ixz"
  Demux1/6 -> Mux/6, Mux/8  "Iyz"
  Mux/1 -> Reshape/1
  Reshape/1 -> inertia/1

== system L400_airframe/force/Mass/For Each Subsystem ==
  note: 惯性张量平移公式
      | Ib = Ia + m*(pab'*pab*eye(3) - pab*pab');
      |
      | Ia是以重心为原点的惯性张量，Ib是移动后的惯性张量
  note: 惯性张量旋转公式
      | Ib = Rab * Ia * Rab'
  Ia : Inport  Partition=on  PartitionDimension=3  PartitionWidth=1  PartitionOffset=0
  m : Inport  Port=2  Partition=on  PartitionDimension=3  PartitionWidth=1  PartitionOffset=0
  pos : Inport  Port=3  Partition=on  PartitionDimension=3  PartitionWidth=1  PartitionOffset=0
  cog : Inport  Port=4
  R : Inport  Port=5
  For Each : ForEach  DisableCoverage=on
  IdentityMatrix : IdentityMatrix  OutputDimensions=3  OutDataTypeStr=Inherit: Inherit via back propagation
  Product : Product  Multiplication=Matrix(*)
  Product1 : Product  Multiplication=Matrix(*)
  Product2 : Product
  Product3 : Product  Inputs=3  Multiplication=Matrix(*)
  Product4 : Product
  Reshape : Reshape
  Sum : Sum  Inputs=|+-
  Sum1 : Sum  Inputs=-+|
  Sum2 : Sum  Inputs=|++
  Transpose : Math  Operator=transpose
  Transpose1 : Math  Operator=transpose
  Ib : Outport  ConcatenationDimension=3
  wires:
  cog/1 -> Sum/2
  pos/1 -> Sum/1
  Ia/1 -> Sum2/2
  Sum/1 -> Reshape/1
  Reshape/1 -> Product1/1, Product/2, Transpose/1
  IdentityMatrix/1 -> Product4/2
  Transpose/1 -> Product1/2, Product/1
  Product1/1 -> Sum1/1
  Sum1/1 -> Product2/1
  m/1 -> Product2/2
  Product2/1 -> Sum2/1
  Sum2/1 -> Product3/2
  R/1 -> Transpose1/1, Product3/1
  Transpose1/1 -> Product3/3
  Product3/1 -> Ib/1
  Product/1 -> Product4/1
  Product4/1 -> Sum1/2

== system L400_airframe/force/Moment/For Each Subsystem ==
  note: 从构型坐标系（后右上）转机体坐标系（前右下）
  Fxyz : Inport  Partition=on  PartitionDimension=2  PartitionWidth=1  PartitionOffset=0
  Mxyz : Inport  Port=2  Partition=on  PartitionDimension=2  PartitionWidth=1  PartitionOffset=0
  Pxyz : Inport  Port=3  Partition=on  PartitionDimension=2  PartitionWidth=1  PartitionOffset=0
  COG : Inport  Port=4
  Cross Product : matrix_library/Cross Product
  For Each : ForEach  DisableCoverage=on
  Gain : Gain  Gain=[-1; 1; -1]
  Sum : Sum  Inputs=|+-
  Sum1 : Sum  Inputs=|++
  M : Outport  ConcatenationDimension=2
  wires:
  Mxyz/1 -> Sum1/2
  Sum/1 -> Gain/1
  Fxyz/1 -> Cross Product/2
  Sum1/1 -> M/1
  Cross Product/1 -> Sum1/1
  COG/1 -> Sum/2
  Gain/1 -> Cross Product/1
  Pxyz/1 -> Sum/1

== system L400_airframe/dynamic/aerodynamic/actuator/Variant Subsystem ==
  note: 1) Add Subsystem or Model blocks as valid variant choices.
      | 2) You cannot connect blocks at this level. At simulation, connectivity is automatically
      | determined, based on the active variant and port name matching.
  In1 : Inport
  Direct Through : Subsystem  VariantControl=true
  Linear : Subsystem  VariantControl=false
  Out1 : Outport

== system L400_airframe/dynamic/aerodynamic/aerodynamics/If Action Subsystem ==
  BusElementIn7 : Inport  PortName=surface
  BusElementIn9 : Inport  Port=2  PortName=state
  BusElementIn1 : Inport  Port=2  PortName=state
  TC : Inport  Port=3
  Action Port : ActionPort  ActionPortLabel=if(u1 > 3)
  CD : Subsystem
  CL : Subsystem
  CM : Subsystem
  CN : Subsystem
  CR : Subsystem
  CY : Subsystem
  Mux2 : Mux  Inputs=3
  Mux3 : Mux  Inputs=3
  Subsystem : Subsystem
  Unary Minus : UnaryMinus
  Unary Minus1 : UnaryMinus
  Bus Element Out : Outport  PortName=aerody
  wires:
  Mux2/1 -> Subsystem/3(CR_CM_CN)  "CR_CM_CN"
  Subsystem/1(aerody) -> Bus Element Out/1
  Unary Minus1/1 -> Mux3/3
  CN/1(CN) -> Mux2/3
  TC/1 -> CL/1(TC), CM/1(TC), CN/1(TC), CR/1(TC), CY/1(TC), CD/1(TC)
  CD/1(CD) -> Unary Minus/1
  CM/1(CM) -> Mux2/2
  CL/1(CL) -> Unary Minus1/1  "CL"
  CY/1(CY) -> Mux3/2
  CR/1(CR) -> Mux2/1
  BusElementIn7/1 -> CM/2(surface), CN/2(surface), CR/2(surface), CL/2(surface), CY/2(surface), CD/2(surface)
  Unary Minus/1 -> Mux3/1
  Mux3/1 -> Subsystem/1(CD_CY_CL)  "CD_CY_CL"
  BusElementIn9/1 -> CR/3(state), CM/3(state), CN/3(state), CL/3(state), CY/3(state), CD/3(state)
  BusElementIn1/1 -> Subsystem/2(state)

== system L400_airframe/dynamic/aerodynamic/aerodynamics/If Action Subsystem1 ==
  Action Port : ActionPort  ActionPortLabel=else
  Constant : Constant  Value=db.aerody.COP
  Constant1 : Constant  Value=[0 0 0]
  Constant2 : Constant  Value=[0 0 0]
  Bus Element Out : Outport  PortName=aerody  Element=Fxyz
  Bus Element Out1 : Outport  PortName=aerody  Element=Mxyz
  Bus Element Out3 : Outport  PortName=aerody  Element=Pxyz
  wires:
  Constant/1 -> Bus Element Out3/1
  Constant2/1 -> Bus Element Out1/1  "aerody_Mxyz"
  Constant1/1 -> Bus Element Out/1

== system L400_airframe/dynamic/landgear/Simple/ground static friction ==
  note: 计算地面静摩擦力
  note: 重心位置（构型系）
  note: 机轮安装位置（构型系）
  Constant1 : Constant  Value=db.landgear.rear_pos
  Constant2 : Constant  Value=db.landgear.right_pos
  Constant3 : Constant  Value=db.landgear.left_pos
  MATLAB Function : MATLAB Function  TreatAsAtomicUnit=on
  Matrix Concatenate3 : Concatenate  NumInputs=3  Mode=Multidimensional array  ConcatenateDimension=2
  Selector : Selector  NumberOfDimensions=2  InputPortWidth=3  IndexOptions=Select all,Index vector (dialog)  Indices=[1 3],1  OutputSizes=1,1
  Selector1 : Selector  NumberOfDimensions=2  InputPortWidth=3  IndexOptions=Select all,Index vector (dialog)  Indices=[1 3],2  OutputSizes=1,1
  Selector2 : Selector  NumberOfDimensions=2  InputPortWidth=3  IndexOptions=Select all,Index vector (dialog)  Indices=[1 3],3  OutputSizes=1,1
  Bus Element Out2 : Outport  PortName=rear  Element=position
  Bus Element Out3 : Outport  PortName=rear  Element=reaction
  Bus Element Out1 : Outport  Port=2  PortName=left  Element=position
  Bus Element Out4 : Outport  Port=2  PortName=left  Element=reaction
  Bus Element Out : Outport  Port=3  PortName=right  Element=position
  Bus Element Out5 : Outport  Port=3  PortName=right  Element=reaction
  wires:
  [Fxyz_no_ground] -> MATLAB Function/1(Fxyz)
  MATLAB Function/1(Fstatic) -> Selector/1, Selector2/1, Selector1/1
  [Mxyz_no_ground] -> MATLAB Function/2(Mxyz)
  Selector/1 -> Bus Element Out3/1
  Selector1/1 -> Bus Element Out4/1
  Selector2/1 -> Bus Element Out5/1
  Constant3/1 -> Bus Element Out1/1, Matrix Concatenate3/2
  [cog] -> MATLAB Function/4(COG)
  Constant1/1 -> Bus Element Out2/1, Matrix Concatenate3/1
  Constant2/1 -> Bus Element Out/1, Matrix Concatenate3/3
  Matrix Concatenate3/1 -> MATLAB Function/3(POS)

== system L400_airframe/dynamic/landgear/Simple/left ==
  note: Pacejka魔术公式是用于轮胎力学特性拟合的经验公式，它由荷兰Delft工业大学H.B. Pacejka与Bakker于1987年提出的半经验轮胎力学模型。
      | 该模型通过三角函数组合公式y = D sin{C arctan[Bx - E(Bx - arctan(Bx))]}，对轮胎试验数据进行回归分析，统一表达纵向力、侧向力、回正力矩等六分力学特性。作为汽车动力学仿真的核心工具，魔术公式被广泛应用于轮胎制造商的数据标准化处理，并在ADAMS、SWIFT等软件中实现操纵稳定性分析。其优势在于突破传统理论模型精度限制，但存在参数与垂直载荷关系需实验获取的局限性。
  note: 转到机体坐标系
  BusElementIn4 : Inport  PortName=cmd
  BusElementIn3 : Inport  Port=2  PortName=state
  Bus Element In4 : Inport  Port=3  PortName=param
  BusElementIn : Inport  Port=3  PortName=param  Element=position
  cog : Inport  Port=4
  Abs : Abs  SaturateOnIntegerOverflow=off
  Bus Selector : BusSelector  OutputSignals=dcm_gear2body
  Bus Selector1 : BusSelector  OutputSignals=wow
  Constant : Constant  Value=[0 0 0]
  Matrix Multiply : Product  Multiplication=Matrix(*)
  Mux1 : Mux  Inputs=3
  Product3 : Product
  侧向摩擦力 : Subsystem
  地面支反力 : Subsystem
  纵向摩擦力 : Subsystem
  计算压缩量 : Subsystem
  Fxyz : Outport
  Mxyz : Outport  Port=2
  Pxyz : Outport  Port=3
  wires:
  Abs/1 -> 侧向摩擦力/2(|Fz|), 纵向摩擦力/2(|Fz|)
  地面支反力/1(Fz) -> Abs/1, Mux1/3
  Mux1/1 -> Matrix Multiply/2
  侧向摩擦力/1(Fy) -> Mux1/2
  纵向摩擦力/1(Fx) -> Mux1/1
  cog/1 -> 计算压缩量/4(cog)
  Bus Element In4/1 -> 计算压缩量/3(param)
  BusElementIn/1 -> Pxyz/1
  Constant/1 -> Mxyz/1
  Bus Selector/1 -> Matrix Multiply/1  "<dcm_gear2body>"
  Matrix Multiply/1 -> Product3/1
  Bus Selector1/1 -> Product3/2  "<wow>"
  Product3/1 -> Fxyz/1
  计算压缩量/1(gear) -> 侧向摩擦力/1(gear), Bus Selector/1, 纵向摩擦力/1(gear), 地面支反力/1(gear), Bus Selector1/1
  BusElementIn3/1 -> 计算压缩量/2(state)
  BusElementIn4/1 -> 计算压缩量/1(cmd)

== system L400_airframe/dynamic/landgear/Simple/rear ==
  note: 转到机体坐标系
  note: Pacejka魔术公式是用于轮胎力学特性拟合的经验公式，它由荷兰Delft工业大学H.B. Pacejka与Bakker于1987年提出的半经验轮胎力学模型。
      | 该模型通过三角函数组合公式y = D sin{C arctan[Bx - E(Bx - arctan(Bx))]}，对轮胎试验数据进行回归分析，统一表达纵向力、侧向力、回正力矩等六分力学特性。作为汽车动力学仿真的核心工具，魔术公式被广泛应用于轮胎制造商的数据标准化处理，并在ADAMS、SWIFT等软件中实现操纵稳定性分析。其优势在于突破传统理论模型精度限制，但存在参数与垂直载荷关系需实验获取的局限性。
  BusElementIn4 : Inport  PortName=cmd
  BusElementIn3 : Inport  Port=2  PortName=state
  Bus Element In4 : Inport  Port=3  PortName=param
  BusElementIn : Inport  Port=3  PortName=param  Element=position
  cog : Inport  Port=4
  Abs : Abs  SaturateOnIntegerOverflow=off
  Bus Selector : BusSelector  OutputSignals=dcm_gear2body
  Bus Selector1 : BusSelector  OutputSignals=wow
  Constant : Constant  Value=[0 0 0]
  Matrix Multiply : Product  Multiplication=Matrix(*)
  Mux1 : Mux  Inputs=3
  Product3 : Product
  侧向摩擦力 : Subsystem
  地面支反力 : Subsystem
  纵向摩擦力 : Subsystem
  计算压缩量 : Subsystem
  Fxyz : Outport
  Mxyz : Outport  Port=2
  Pxyz : Outport  Port=3
  wires:
  BusElementIn4/1 -> 计算压缩量/1(cmd)
  BusElementIn3/1 -> 计算压缩量/2(state)
  计算压缩量/1(gear) -> Bus Selector1/1, 地面支反力/1(gear), 纵向摩擦力/1(gear), Bus Selector/1, 侧向摩擦力/1(gear)
  Product3/1 -> Fxyz/1
  Bus Selector1/1 -> Product3/2  "<wow>"
  Matrix Multiply/1 -> Product3/1
  Bus Selector/1 -> Matrix Multiply/1  "<dcm_gear2body>"
  Constant/1 -> Mxyz/1
  BusElementIn/1 -> Pxyz/1
  Bus Element In4/1 -> 计算压缩量/3(param)
  cog/1 -> 计算压缩量/4(cog)
  纵向摩擦力/1(Fx) -> Mux1/1
  侧向摩擦力/1(Fy) -> Mux1/2
  Mux1/1 -> Matrix Multiply/2
  地面支反力/1(Fz) -> Mux1/3, Abs/1
  Abs/1 -> 纵向摩擦力/2(|Fz|), 侧向摩擦力/2(|Fz|)

== system L400_airframe/dynamic/landgear/Simple/right ==
  note: 转到机体坐标系
  note: Pacejka魔术公式是用于轮胎力学特性拟合的经验公式，它由荷兰Delft工业大学H.B. Pacejka与Bakker于1987年提出的半经验轮胎力学模型。
      | 该模型通过三角函数组合公式y = D sin{C arctan[Bx - E(Bx - arctan(Bx))]}，对轮胎试验数据进行回归分析，统一表达纵向力、侧向力、回正力矩等六分力学特性。作为汽车动力学仿真的核心工具，魔术公式被广泛应用于轮胎制造商的数据标准化处理，并在ADAMS、SWIFT等软件中实现操纵稳定性分析。其优势在于突破传统理论模型精度限制，但存在参数与垂直载荷关系需实验获取的局限性。
  BusElementIn4 : Inport  PortName=cmd
  BusElementIn3 : Inport  Port=2  PortName=state
  Bus Element In4 : Inport  Port=3  PortName=param
  BusElementIn : Inport  Port=3  PortName=param  Element=position
  cog : Inport  Port=4
  Abs : Abs  SaturateOnIntegerOverflow=off
  Bus Selector : BusSelector  OutputSignals=dcm_gear2body
  Bus Selector1 : BusSelector  OutputSignals=wow
  Constant : Constant  Value=[0 0 0]
  Matrix Multiply : Product  Multiplication=Matrix(*)
  Mux1 : Mux  Inputs=3
  Product3 : Product
  侧向摩擦力 : Subsystem
  地面支反力 : Subsystem
  纵向摩擦力 : Subsystem
  计算压缩量 : Subsystem
  Fxyz : Outport
  Mxyz : Outport  Port=2
  Pxyz : Outport  Port=3
  wires:
  BusElementIn4/1 -> 计算压缩量/1(cmd)
  BusElementIn3/1 -> 计算压缩量/2(state)
  计算压缩量/1(gear) -> Bus Selector1/1, 地面支反力/1(gear), 纵向摩擦力/1(gear), Bus Selector/1, 侧向摩擦力/1(gear)
  Product3/1 -> Fxyz/1
  Bus Selector1/1 -> Product3/2  "<wow>"
  Matrix Multiply/1 -> Product3/1
  Bus Selector/1 -> Matrix Multiply/1  "<dcm_gear2body>"
  Constant/1 -> Mxyz/1
  BusElementIn/1 -> Pxyz/1
  Bus Element In4/1 -> 计算压缩量/3(param)
  cog/1 -> 计算压缩量/4(cog)
  纵向摩擦力/1(Fx) -> Mux1/1
  侧向摩擦力/1(Fy) -> Mux1/2
  Mux1/1 -> Matrix Multiply/2
  地面支反力/1(Fz) -> Mux1/3, Abs/1
  Abs/1 -> 纵向摩擦力/2(|Fz|), 侧向摩擦力/2(|Fz|)
